simulink model "SS_Part5"  (R2024b)
settings: Solver=FixedStepAuto  StartTime=0.0  StopTime=tspan  FixedStep=10  RelTol=1e-3
values from neighbouring files (symbols this model uses):
  Eul0_b_eci = Eul0_b_eci(:)    [Final_3.m]    (also in ORR_part4_script.m = [phi_b_eci_0; theta_b_eci_0; psi_b_eci_0]; Part2_TorqueFreeMotion.m = [phi_b_eci_0; theta_b_eci_0; psi_b_eci_0]; Part2_TorqueFreeMotion_SS.m = [phi_b_eci_0; theta_b_eci_0; psi_b_eci_0]; Part5_TorqueFreeMotion_SS.m = [phi_b_eci_0; theta_b_eci_0; psi_b_eci_0])
  Kd = J/ts    [Part5_TorqueFreeMotion_SS.m]    (also in Part_5_ORR.m = J*eye(3)*2*zeta*wn; SS_Part6Script.m = 2*zeta*wn*I_tot)
  Kp = zeros(3)    [Part5_TorqueFreeMotion_SS.m]    (also in Part_5_ORR.m = 2*J*eye(3)*wn^2; SS_Part6Script.m = 2*wn^2*I_tot)
  q0_b_eci = q0_b_eci(:)    [Final_3.m]    (also in ORR_part4_script.m; Part2_TorqueFreeMotion.m = DCM_to_quat(C_b_ECI_0); Part2_TorqueFreeMotion_SS.m = DCM_to_quat(C_b_ECI_0); Part5_TorqueFreeMotion_SS.m = DCM_to_quat(C_b_ECI_0))
  q_C = [0; 0; 0; 1]    [Part5_TorqueFreeMotion_SS.m]    (also in SS_Part6Script.m = [0;0;0;1])
  w0_b_eci = [0.001; -0.001; 0.002]    [Part2_TorqueFreeMotion.m]    (also in Part2_TorqueFreeMotion_SS.m; Part5_TorqueFreeMotion_SS.m)
undefined symbols (not defined in the file or in its folder): n
settings Model: Creator=emehiel  LastModifiedBy=dstan
settings SolverCC: AlgebraicLoopSolver=TrustRegion
settings DebuggingCC: UnconnectedInputMsg=warning  UnconnectedOutputMsg=warning  UnconnectedLineMsg=warning
settings ModelReferenceCC: EnableRefExpFcnMdlSchedulingChecks=on
settings RTWCC: GPUComputeCapability=3.5

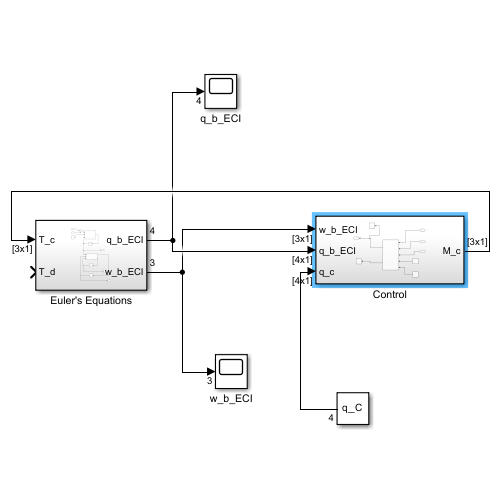
[thumbnail: Simulink's stored preview of the top-level diagram]
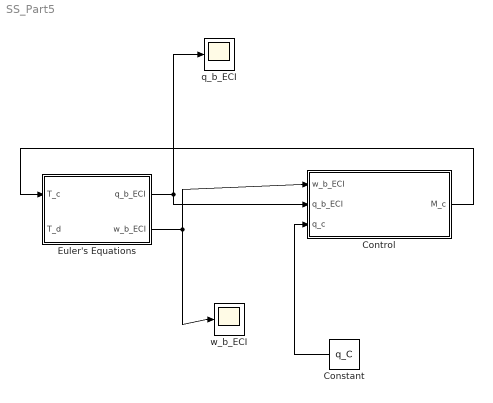
== system SS_Part5 ==
  Constant : Constant  Value=q_C
  Control : Subsystem
  Euler's Equations : Subsystem
  q_b_ECI : Scope
  w_b_ECI : Scope
  wires:
  Euler's Equations/1(q_b_ECI) -> q_b_ECI/1, Control/2(q_b_ECI)
  Euler's Equations/2(w_b_ECI) -> w_b_ECI/1, Control/1(w_b_ECI)
  Constant/1 -> Control/3(q_c)
  Control/1(M_c) -> Euler's Equations/1(T_c)

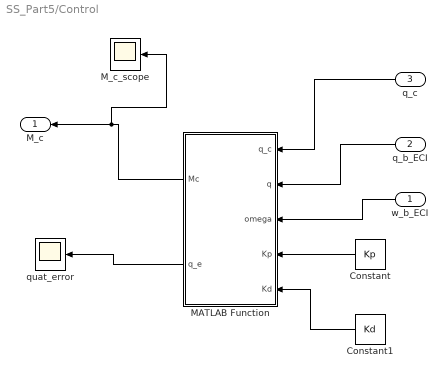
== system SS_Part5/Control ==
  w_b_ECI : Inport  PortDimensions=[3 1]
  q_b_ECI : Inport  Port=2  PortDimensions=[4 1]
  q_c : Inport  Port=3  PortDimensions=[4 1]
  Constant : Constant  Value=Kp
  Constant1 : Constant  Value=Kd
  MATLAB Function : MATLAB Function  TreatAsAtomicUnit=on
  M_c_scope : Scope
  quat_error : Scope
  M_c : Outport  PortDimensions=[3 1]  VectorParamsAs1DForOutWhenUnconnected=off
  wires:
  MATLAB Function/1(Mc) -> M_c_scope/1, M_c/1
  q_c/1 -> MATLAB Function/1(q_c)
  w_b_ECI/1 -> MATLAB Function/3(omega)
  q_b_ECI/1 -> MATLAB Function/2(q)
  Constant/1 -> MATLAB Function/4(Kp)
  MATLAB Function/2(q_e) -> quat_error/1
  Constant1/1 -> MATLAB Function/5(Kd)

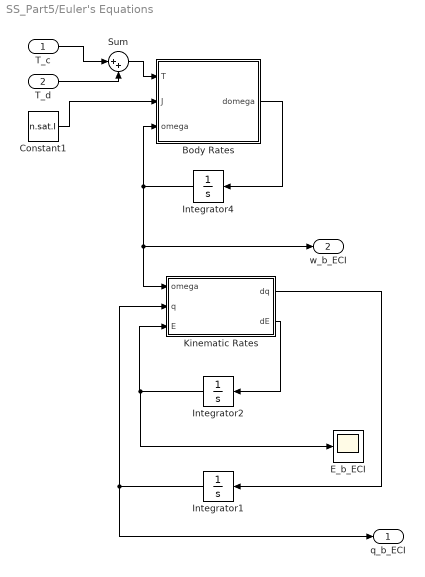
== system SS_Part5/Euler's Equations ==
  T_c : Inport
  T_d : Inport  Port=2
  Body Rates : MATLAB Function  TreatAsAtomicUnit=on
  Constant1 : Constant  Value=n.sat.I
  E_b_ECI : Scope
  Integrator1 : Integrator  InitialCondition=q0_b_eci  AbsoluteTolerance=1e-10
  Integrator2 : Integrator  InitialCondition=Eul0_b_eci
  Integrator4 : Integrator  InitialCondition=w0_b_eci
  Kinematic Rates : MATLAB Function  TreatAsAtomicUnit=on
  Sum : Sum  Inputs=|++
  q_b_ECI : Outport
  w_b_ECI : Outport  Port=2
  wires:
  Integrator4/1 -> Body Rates/3(omega), w_b_ECI/1, Kinematic Rates/1(omega)
  Integrator2/1 -> E_b_ECI/1, Kinematic Rates/3(E)
  Kinematic Rates/1(dq) -> Integrator1/1
  Integrator1/1 -> q_b_ECI/1, Kinematic Rates/2(q)
  Body Rates/1(domega) -> Integrator4/1
  Constant1/1 -> Body Rates/2(J)
  Kinematic Rates/2(dE) -> Integrator2/1
  Sum/1 -> Body Rates/1(T)
  T_c/1 -> Sum/1
  T_d/1 -> Sum/2

== matlab function SS_Part5/Euler's Equations/Kinematic Rates ==
  data: omega input; q input; dq output; E input; dE output
function [dq, dE] = kinematics(omega, q, E)
% column vecs
omega = omega(:);
q = q(:);
E = E(:);

% unpack euler angles
phi = E(1);
theta = E(2);
psi = E(3);

% unpack quat
eps = q(1:3);
eta = q(4);

% euler derivative
B = [1, sin(phi)*tan(theta),  cos(phi)*tan(theta);
     0, cos(phi),            -sin(phi);
     0, sin(phi)/cos(theta),  cos(phi)/cos(theta)];

dE = B * omega;

% quat derivative
dq = zeros(4,1);
dq(1:3) = 0.5 * ((eta*eye(3) + skew(eps)) * omega);
dq(4)   = -0.5 * (eps.' * omega);

end

== matlab function SS_Part5/Euler's Equations/Body Rates ==
  data: T input; J input; omega input; domega output
function domega = dynamics(T, J, omega)

%column vecs
omega = omega(:);
T = T(:);

domega = J \ (T - cross(omega, J*omega));
end

== matlab function SS_Part5/Control/MATLAB Function ==
  data: q_c input; Mc output; q input; omega input; Kp input; Kd input; q_e output
function [Mc,q_e]  = control_law(q_c, q, omega, Kp, Kd)
%#codegen

q_e = quatMult(q, quatConjugate(q_c));
%Mc = -Kp*q_e(1:3,1) - Kd*omega;
% Only detumble
Mc = -Kd*omega;
